simulink model "BlockDemo2"  (Simulink 6.3)
settings: Solver=ode45  StartTime=0.0  StopTime=10.0  RelTol=1e-3
InitFcn:
  | %% DSPBuilder Start
  | alt_dspbuilder_update_model(bdroot)
  | %% DSPBuilder End
libraries: allblocks_alteradspbuilder2 x4
settings Model: LastModifiedBy=delphick
settings OptimizationCC: BooleanDataType=off  InlineInvariantSignals=on
settings DebuggingCC: SolverPrmCheckMsg=none
settings HardwareCC: TargetUnknown=on

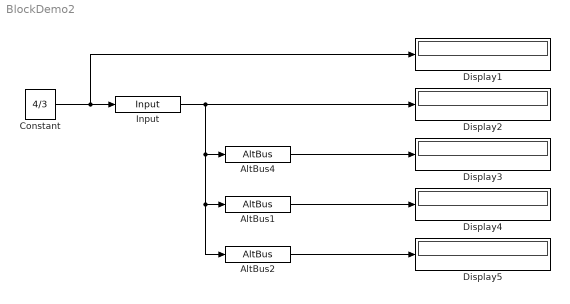
== system BlockDemo2 ==
  AltBus1 : allblocks_alteradspbuilder2/AltBus  BusType=Signed Fractional  bwl=2  bwr=5  saturate=off
  AltBus2 : allblocks_alteradspbuilder2/AltBus  BusType=Signed Fractional  bwl=2  bwr=8  saturate=off
  AltBus4 : allblocks_alteradspbuilder2/AltBus  BusType=Signed Fractional  bwl=2  bwr=2  saturate=off
  Constant : Constant  Value=4/3
  Display{1..5} (5 alike) : Display
  Input : allblocks_alteradspbuilder2/Input  iofile=C:\workspace_clean\Documentation\DesignExamples\Tutorials\UnitBlocks\IOBus\AltBus\tb_BlockDemo2\BlockDemo2_Input.salt  BusType=Signed Fractional  bwl=10  bwr=10  SpecifyClock=off  PORTTYPE=Input
  wires:
  Constant/1 -> Input/1, Display1/1
  Input/1 -> AltBus1/1, AltBus2/1, AltBus4/1, Display2/1
  AltBus2/1 -> Display5/1
  AltBus1/1 -> Display4/1
  AltBus4/1 -> Display3/1
